simulink model "krzywe"  (R2022b)
settings: Solver=ode4  StartTime=0.0  StopTime=10.0  FixedStep=0.1  RelTol=1e-3
settings Model: Creator=karol  LastModifiedBy=karol

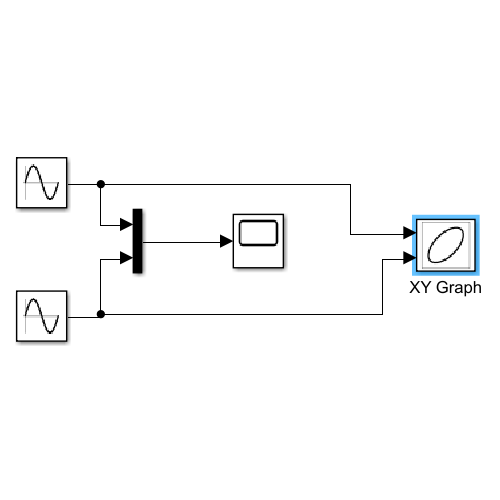
[thumbnail: Simulink's stored preview of the top-level diagram]
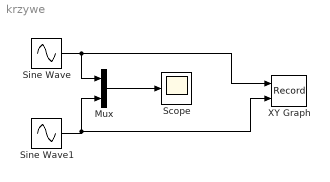
== system krzywe ==
  Mux : Mux  Inputs=2
  Scope : Scope
  Sine Wave : Sin  Frequency=3  SampleTime=0
  Sine Wave1 : Sin  Frequency=2  SampleTime=0
  XY Graph : Record  FileSettingsInternal="{\"entries\":[{\"content\":{\"excelSettings\":{\"content\":{},\"type\":\"Streamout.ExcelSettings\"}},\"type\":\"Streamout.FileSettingStorage\",\"uuid\":\"68455f09-34b2-4409-b37d-96a1d2ab39fb\"}],\"packageUris\":[\"http://schema.mathworks.com/mf0/streamout_blocks/R2020a\"],\"version\":\"1.0\"}"  Layout=[1 1]  SignalsInternal="{\"entries\":[{\"content\":{\"signals\":[{\"content\":{\"blockPath\":[\"krzywe/XY Graph\"],\"channel\":[],\"dimensions\":[1],\"domain\":\"krzywe/XY Graph\",\"lineColor\":\"#a2142f\",\"plots\":[1],\"port\":1,\"sid\":[\"\"],\"signalID\":251,\"signalName\":\"Sine Wave\"},\"type\":\"RecordBlkView.Signal\",\"uuid\":\"85cb1a12-efc4-43ca-863b-9da76958a99e\"},{\"content\":{\"blockPath\":[\"krzywe/XY Graph\"],\"channel\":[],\"dimensions\":[1],\"domain\":\"krzywe/XY Graph\",\"lineColor\":\"#139fff\",\"plots\":[1],\"port\":2,\"sid\":[\"\"],\"signalID\":255,\"signalName\":\"Sine Wave1\"},\"type\":\"RecordBlkView.Signal\",\"uuid\":\"8bc35672-9307-4315-a70c-fee54fd5fd3a\"}]},\"type\":\"RecordBlkView.InputSignals\",\"uuid\":\"32c58755-4980-4ed7-81f0-e78c3e87ac10\"}],\"packageUris\":[\"http://schema.mathworks.com/mf0/streamout_blocks/R2020a\"],\"version\":\"1.0\"}"  VisualizationBindings="{\"xyplotplugin\":{\"info\":[{\"series\":[{\"bindingParametersList\":[{\"parameter\":\"X-Axis\",\"signalID\":251,\"signalName\":\"Sine Wave\"},{\"parameter\":\"Y-Axis\",\"signalID\":255,\"signalName\":\"Sine Wave1\"}],\"seriesID\":48944}],\"subplotID\":1}]}}"  CompatibilityTag=XY
  wires:
  Mux/1 -> Scope/1
  Sine Wave/1 -> XY Graph/1, Mux/1
  Sine Wave1/1 -> XY Graph/2, Mux/2
